simulink model "Final_Project_2_test"  (R2023b)
settings: Solver=FixedStepAuto  StartTime=0.0  StopTime=inf  FixedStep=0.01  RelTol=1e-3  EnableMultiTasking=on
libraries: arduinolib x9, arduinosensorlib x1
settings Model: ExtModeTrigDuration=2  Creator=FM23  LastModifiedBy=FM23
settings OptimizationCC: EnhancedBackFolding=on  PassReuseOutputArgsAs=Individual arguments  ZeroExternalMemoryAtStartup=off  ZeroInternalMemoryAtStartup=off  MaxStackSize=64  OptimizeBlockOrder=speed  DifferentSizesBufferReuse=on  OptimizationCustomize=off  EfficientTunableParamExpr=on
settings DebuggingCC: ParameterTunabilityLossMsg=error
settings HardwareCC: ProdBitPerInt=16  ProdBitPerPointer=16  ProdBitPerSizeT=16  ProdBitPerPtrDiffT=16  ProdLargestAtomicFloat=None  ProdWordSize=8  ProdHWDeviceType=Atmel->AVR
settings SFSimCC: MATLABDynamicMemAlloc=off
settings RTWCC: Description=Embedded Coder  SystemTargetFile=ert.tlc  HardwareBoard=Arduino Mega 2560  TemplateMakefile=ert_default_tmf  Toolchain=Arduino AVR  BuildConfiguration=Faster Runs
settings CodeAppCC: ForceParamTrailComments=on  IgnoreCustomStorageClasses=off  OperatorAnnotations=on  SimulinkDataObjDesc=on  SFDataObjDesc=on  InsertBlockDesc=on
settings ERTTargetCC: SupportContinuousTime=on  SupportVariableSizeSignals=on  ExtModeTransport=3  ExtModeStaticAlloc=on  ExtModeAutomaticAllocSize=off  ExtModeStaticAllocSize=2048  ExtModeMexFile=ext_xcp  ExtModeIntrfLevel=Level2 - Open

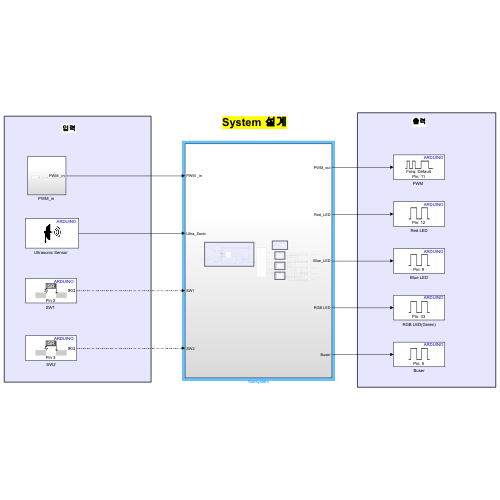
[thumbnail: Simulink's stored preview of the top-level diagram]
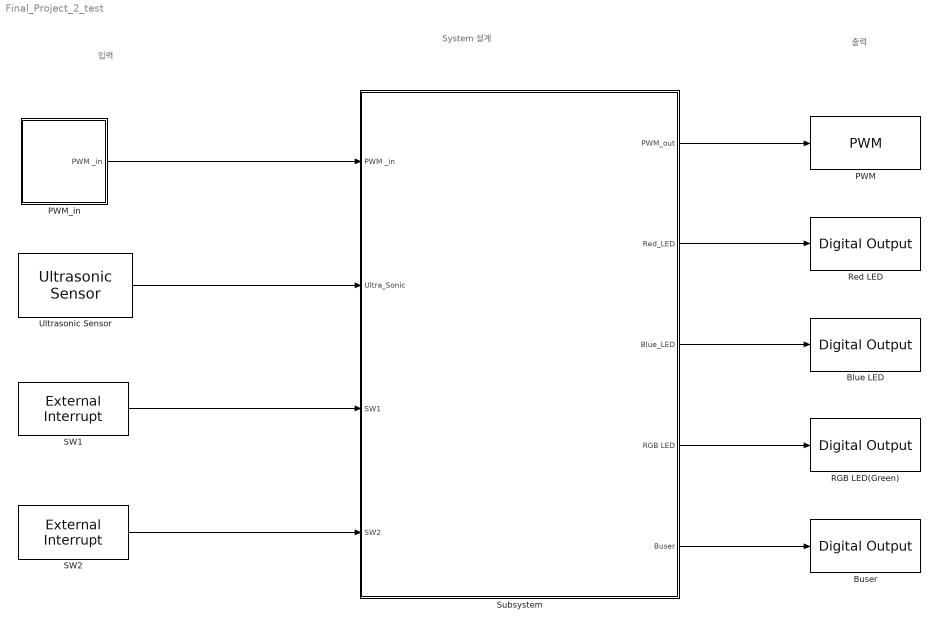
== system Final_Project_2_test ==
  note: System 설계
  note: 입력
  note: 출력
  Blue LED : arduinolib/Digital Output  pinNumber=9  Direction=output  blockPlatform=arduino
  Buser : arduinolib/Digital Output  pinNumber=5  Direction=output  blockPlatform=arduino
  "PWM  " : arduinolib/PWM  pinNumber=11  frequencyType=Default  desiredFrequency=490.2  achievableFrequency=490.2
  "PWM_in " : Subsystem
  RGB LED(Green) : arduinolib/Digital Output  pinNumber=33  Direction=output  blockPlatform=arduino
  Red LED : arduinolib/Digital Output  pinNumber=12  Direction=output  blockPlatform=arduino
  "SW1 " : arduinolib/External Interrupt  Pin=2  PullUp=off  Mode=RISING  InterruptSimulationInput=off
  SW2 : arduinolib/External Interrupt  Pin=3  PullUp=off  Mode=RISING  InterruptSimulationInput=off
  Subsystem : Subsystem
  "Ultrasonic Sensor  " : arduinosensorlib/Ultrasonic Sensor  NumSignalPins=2  TrigPin=50  EchoPin=51  SignalPin=3  SampleTime_=0.01  blockPlatform=ARDUINO
  wires:
  Subsystem/1(" PWM_out") -> "PWM  "/1
  Subsystem/2(Red_LED) -> Red LED/1
  Subsystem/3(Blue_LED) -> Blue LED/1
  "PWM_in "/1(PWM _in) -> Subsystem/1(PWM _in)
  "SW1 "/1 -> Subsystem/3(SW1)
  SW2/1 -> Subsystem/4(SW2)
  "Ultrasonic Sensor  "/1 -> Subsystem/2(Ultra_Sonic)
  Subsystem/4(RGB LED) -> RGB LED(Green)/1
  Subsystem/5(Buser) -> Buser/1

== system Final_Project_2_test/PWM_in  ==
  Analog Input1 : arduinolib/Analog Input  pinNumber=4  ReadResultsOnly=off  ConversionTriggerSource=Software  ExternalTriggerType=uint32( 0 )  OutputDataType=uint16  EnableConversionCompleteNotify=off  EnableOuputStatus=off  SampleTime=-1  blockPlatform=arduino
  Data Type Conversion : DataTypeConversion  OutDataTypeStr=uint8  SaturateOnIntegerOverflow=off  RndMeth=Floor
  Display Status : Display
  Gain : Gain  Gain=0.25
  PWM _in : Outport
  wires:
  Analog Input1/1 -> Gain/1
  Gain/1 -> Data Type Conversion/1
  Data Type Conversion/1 -> PWM _in/1, Display Status/1

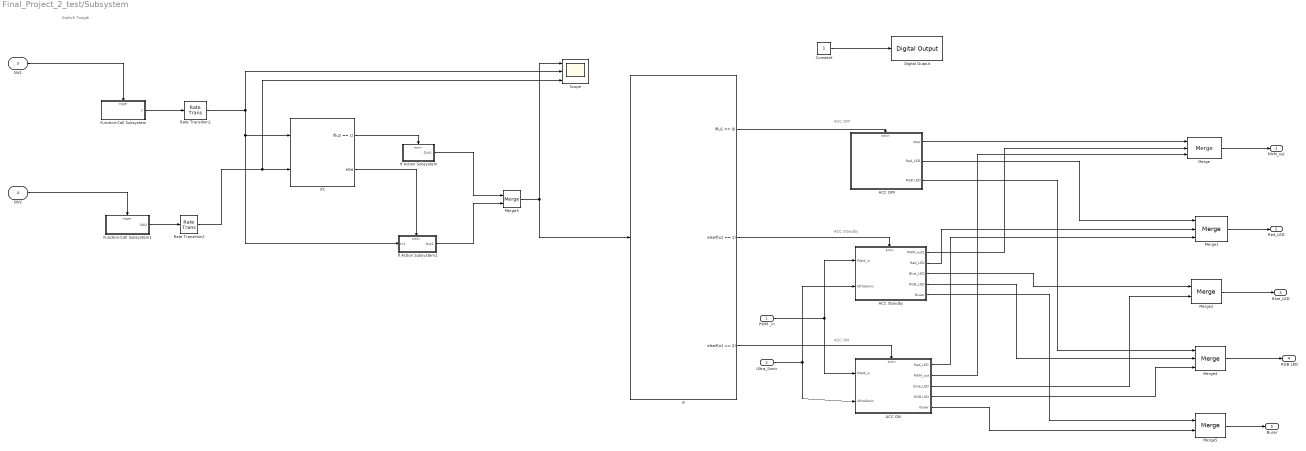
== system Final_Project_2_test/Subsystem ==
  note: ACC ON
  note: ACC standby
  note: ACC OFF
  note: Swiitch Toogle
  PWM _in : Inport
  Ultra_Sonic : Inport  Port=2
  SW1 : Inport  Port=3
  SW2 : Inport  Port=4
  ACC OFF : Subsystem  TreatAsAtomicUnit=on
  ACC ON : Subsystem  TreatAsAtomicUnit=on
  "ACC Standby   " : Subsystem  TreatAsAtomicUnit=on
  Constant : Constant
  Digital Output : arduinolib/Digital Output  pinNumber=13  Direction=output  blockPlatform=arduino
  Function-Call Subsystem : Subsystem  TreatAsAtomicUnit=on
  Function-Call Subsystem1 : Subsystem  TreatAsAtomicUnit=on
  If : If  IfExpression=u1 == 0  ElseIfExpressions=u1 == 1, u1 == 2  ShowElse=off
  If Action Subsystem : Subsystem  TreatAsAtomicUnit=on
  If Action Subsystem1 : Subsystem  TreatAsAtomicUnit=on
  If1 : If  NumInputs=2  IfExpression=u2 == 1
  Merge : Merge  Inputs=3
  Merge1 : Merge  Inputs=3
  Merge2 : Merge
  Merge3 : Merge
  Merge4 : Merge  Inputs=3
  Merge5 : Merge
  Rate Transition1 : RateTransition  Integrity=off
  Rate Transition2 : RateTransition  Integrity=off
  Scope : Scope  NumInputPorts=3
  " PWM_out" : Outport
  Red_LED : Outport  Port=2
  Blue_LED : Outport  Port=3
  RGB LED : Outport  Port=4
  Buser : Outport  Port=5
  wires:
  Function-Call Subsystem/1(y) -> Rate Transition1/1
  "ACC Standby   "/1(PWM_out2) -> Merge/2
  "ACC Standby   "/3(Blue_LED) -> Merge2/1
  If/1 -> ACC OFF/Action
  ACC ON/2(PWM_out) -> Merge/3
  ACC OFF/2(Red_LED) -> Merge1/1
  Ultra_Sonic/1 -> "ACC Standby   "/2(UltraSonic), ACC ON/2(UltraSonic)
  Rate Transition1/1 -> If Action Subsystem1/1(In1), If1/1, Scope/2
  SW1/1 -> Function-Call Subsystem/Trigger
  If/3 -> ACC ON/Action
  Merge/1 -> " PWM_out"/1
  "ACC Standby   "/2(Red_LED) -> Merge1/2
  PWM _in/1 -> "ACC Standby   "/1(PWM_in), ACC ON/1(PWM_in)
  Constant/1 -> Digital Output/1
  Merge2/1 -> Blue_LED/1
  If Action Subsystem/1(Out1) -> Merge3/1
  If1/2 -> If Action Subsystem1/Action
  ACC OFF/1(stop) -> Merge/1
  SW2/1 -> Function-Call Subsystem1/Trigger
  If Action Subsystem1/1(Out1) -> Merge3/2
  Function-Call Subsystem1/1(SW2) -> Rate Transition2/1
  Merge1/1 -> Red_LED/1
  Rate Transition2/1 -> Scope/3, If1/2
  Merge3/1 -> Scope/1, If/1
  If1/1 -> If Action Subsystem/Action
  ACC ON/3(Blue_LED) -> Merge2/2
  ACC ON/1(Red_LED) -> Merge1/3
  If/2 -> "ACC Standby   "/Action
  ACC OFF/3(RGB LED) -> Merge4/1
  "ACC Standby   "/4(RGB_LED) -> Merge4/2
  ACC ON/4(RGB LED) -> Merge4/3
  Merge4/1 -> RGB LED/1
  "ACC Standby   "/5(Buser) -> Merge5/1
  ACC ON/5(Buser) -> Merge5/2
  Merge5/1 -> Buser/1

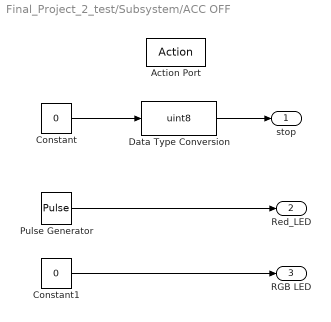
== system Final_Project_2_test/Subsystem/ACC OFF ==
  Action Port : ActionPort  ActionPortLabel=if(u1 == 0)
  Constant : Constant  Value=0
  Constant1 : Constant  Value=0
  Data Type Conversion : DataTypeConversion  OutDataTypeStr=uint8  SaturateOnIntegerOverflow=off  RndMeth=Floor
  Pulse Generator : DiscretePulseGenerator  PulseType=Time based  Period=0.4  PulseWidth=50
  stop : Outport
  Red_LED : Outport  Port=2
  RGB LED : Outport  Port=3
  wires:
  Pulse Generator/1 -> Red_LED/1
  Constant/1 -> Data Type Conversion/1
  Data Type Conversion/1 -> stop/1
  Constant1/1 -> RGB LED/1

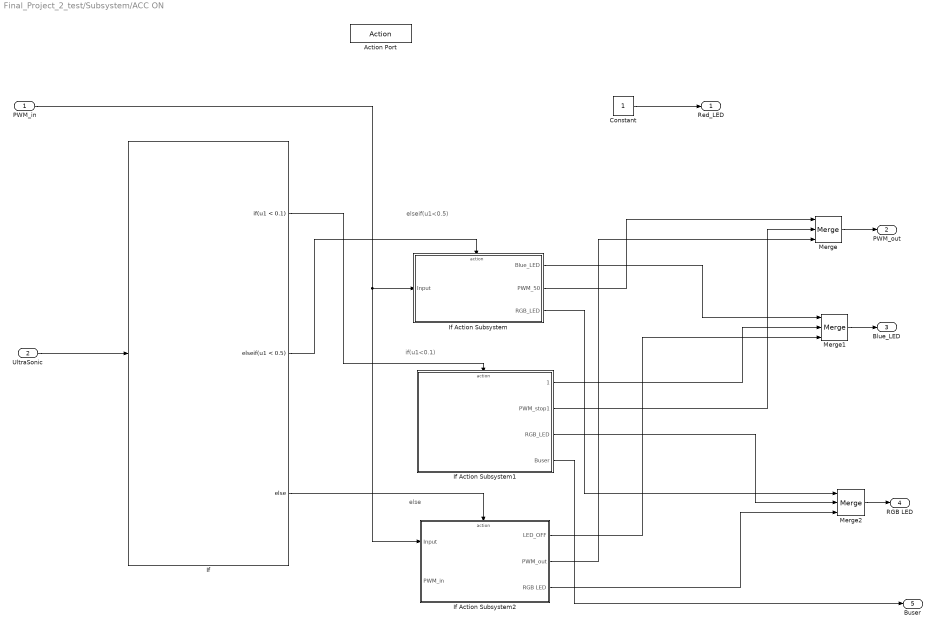
== system Final_Project_2_test/Subsystem/ACC ON ==
  note: if(u1<0.1)
  note: elseif(u1<0.5)
  note: else
  PWM_in : Inport
  UltraSonic : Inport  Port=2
  Action Port : ActionPort  ActionPortLabel=elseif( u1 == 2)
  Constant : Constant
  If : If  IfExpression=u1 < 0.1  ElseIfExpressions=u1 < 0.5
  If Action Subsystem : Subsystem  TreatAsAtomicUnit=on
  If Action Subsystem1 : Subsystem  TreatAsAtomicUnit=on
  If Action Subsystem2 : Subsystem  TreatAsAtomicUnit=on
  Merge : Merge  Inputs=3
  Merge1 : Merge  Inputs=3
  Merge2 : Merge  Inputs=3
  Red_LED : Outport
  PWM_out : Outport  Port=2  OutDataTypeStr=uint8
  Blue_LED : Outport  Port=3
  RGB LED : Outport  Port=4
  Buser : Outport  Port=5
  wires:
  If Action Subsystem2/1(LED_OFF) -> Merge1/3
  If Action Subsystem1/2(PWM_stop1) -> Merge/2
  If Action Subsystem2/2(PWM_out) -> Merge/3
  Merge1/1 -> Blue_LED/1
  If Action Subsystem/1(Blue_LED) -> Merge1/1
  If/2 -> If Action Subsystem/Action
  If/3 -> If Action Subsystem2/Action
  If Action Subsystem1/1(1) -> Merge1/2
  If Action Subsystem/2(PWM_50) -> Merge/1
  If/1 -> If Action Subsystem1/Action
  UltraSonic/1 -> If/1
  Merge/1 -> PWM_out/1
  Constant/1 -> Red_LED/1
  PWM_in/1 -> If Action Subsystem2/1(Input), If Action Subsystem/1(Input)
  If Action Subsystem/3(RGB_LED) -> Merge2/1
  If Action Subsystem1/3(RGB_LED) -> Merge2/2
  If Action Subsystem2/3(RGB LED) -> Merge2/3
  Merge2/1 -> RGB LED/1
  If Action Subsystem1/4(Buser) -> Buser/1

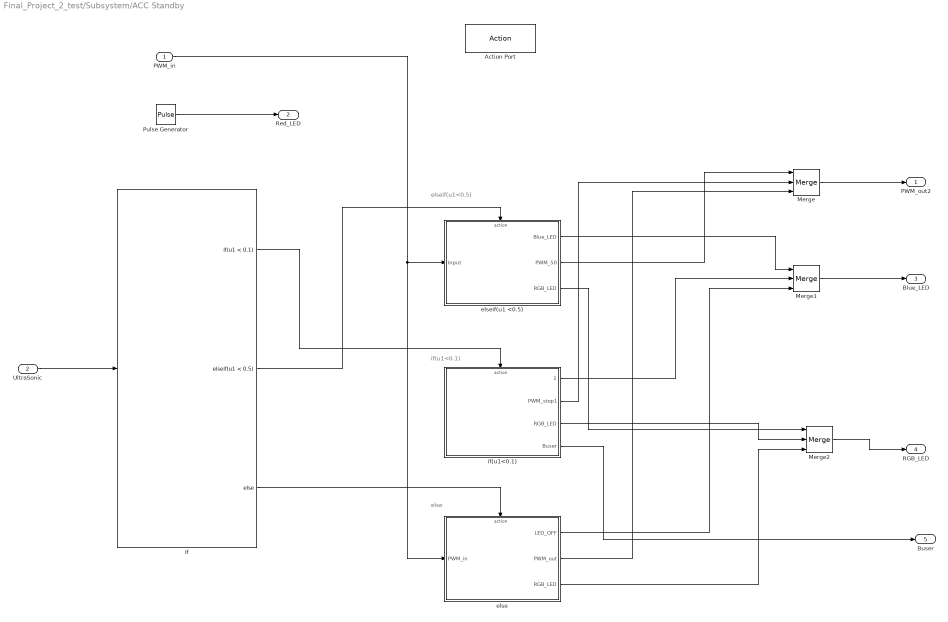
== system Final_Project_2_test/Subsystem/ACC Standby    ==
  note: else
  note: if(u1<0.1)
  note: elseif(u1<0.5)
  PWM_in : Inport  OutDataTypeStr=uint8
  UltraSonic : Inport  Port=2
  Action Port : ActionPort  ActionPortLabel=elseif(u1 == 1)
  If : If  IfExpression=u1 < 0.1  ElseIfExpressions=u1 < 0.5
  Merge : Merge  Inputs=3
  Merge1 : Merge  Inputs=3
  Merge2 : Merge  Inputs=3
  Pulse Generator : DiscretePulseGenerator  PulseType=Time based  Period=10  PulseWidth=5
  else : Subsystem  TreatAsAtomicUnit=on
  elseif(u1 <0.5) : Subsystem  TreatAsAtomicUnit=on
  if(u1<0.1) : Subsystem  TreatAsAtomicUnit=on
  PWM_out2 : Outport
  Red_LED : Outport  Port=2
  Blue_LED : Outport  Port=3
  RGB_LED : Outport  Port=4
  Buser : Outport  Port=5
  wires:
  Pulse Generator/1 -> Red_LED/1
  UltraSonic/1 -> If/1
  Merge/1 -> PWM_out2/1
  Merge1/1 -> Blue_LED/1
  If/2 -> elseif(u1 <0.5)/Action
  If/1 -> if(u1<0.1)/Action
  If/3 -> else/Action
  else/2(PWM_out) -> Merge/3
  elseif(u1 <0.5)/2(PWM_50) -> Merge/1
  elseif(u1 <0.5)/1(Blue_LED) -> Merge1/1
  if(u1<0.1)/1(1) -> Merge1/2
  if(u1<0.1)/2(PWM_stop1) -> Merge/2
  else/1(LED_OFF) -> Merge1/3
  PWM_in/1 -> else/1(PWM_in), elseif(u1 <0.5)/1(Input)
  elseif(u1 <0.5)/3(RGB_LED) -> Merge2/1
  if(u1<0.1)/3(RGB_LED) -> Merge2/2
  else/3(RGB_LED) -> Merge2/3
  Merge2/1 -> RGB_LED/1
  if(u1<0.1)/4(Buser) -> Buser/1

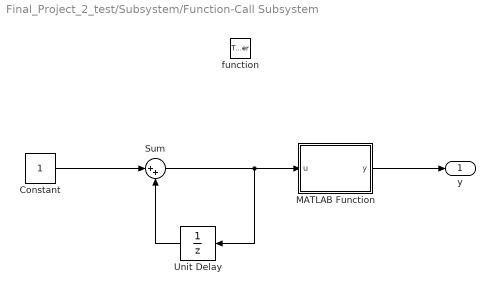
== system Final_Project_2_test/Subsystem/Function-Call Subsystem ==
  function : TriggerPort  TriggerType=function-call  VariantControl=(inherit)
  Constant : Constant
  MATLAB Function : MATLAB Function  TreatAsAtomicUnit=on
  Sum : Sum  Inputs=|++
  Unit Delay : UnitDelay  SampleTime=-1  HasFrameUpgradeWarning=on
  y : Outport
  wires:
  Constant/1 -> Sum/1
  Unit Delay/1 -> Sum/2
  Sum/1 -> Unit Delay/1, MATLAB Function/1(u)
  MATLAB Function/1(y) -> y/1

== system Final_Project_2_test/Subsystem/Function-Call Subsystem1 ==
  function : TriggerPort  TriggerType=function-call  VariantControl=(inherit)
  Constant : Constant
  MATLAB Function : MATLAB Function  TreatAsAtomicUnit=on
  Sum : Sum  Inputs=|++
  Unit Delay : UnitDelay  SampleTime=-1  HasFrameUpgradeWarning=on
  SW2 : Outport
  wires:
  Constant/1 -> Sum/1
  MATLAB Function/1(y) -> SW2/1
  Unit Delay/1 -> Sum/2
  Sum/1 -> Unit Delay/1, MATLAB Function/1(u)

== system Final_Project_2_test/Subsystem/If Action Subsystem ==
  Action Port : ActionPort  ActionPortLabel=if(u2 == 1)
  Constant : Constant  Value=0
  Out1 : Outport
  wires:
  Constant/1 -> Out1/1

== system Final_Project_2_test/Subsystem/If Action Subsystem1 ==
  In1 : Inport
  Action Port : ActionPort  ActionPortLabel=else
  Out1 : Outport
  wires:
  In1/1 -> Out1/1

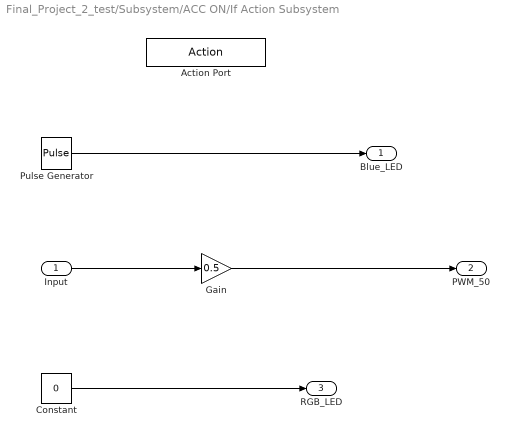
== system Final_Project_2_test/Subsystem/ACC ON/If Action Subsystem ==
  Input : Inport  OutDataTypeStr=uint8
  Action Port : ActionPort  ActionPortLabel=elseif(u1 < 0.5)
  Constant : Constant  Value=0  OutDataTypeStr=double
  Gain : Gain  Gain=0.5  OutDataTypeStr=uint8
  Pulse Generator : DiscretePulseGenerator  PulseType=Time based  Period=0.4  PulseWidth=50
  Blue_LED : Outport
  PWM_50 : Outport  Port=2  OutDataTypeStr=uint8
  RGB_LED : Outport  Port=3  OutDataTypeStr=double
  wires:
  Input/1 -> Gain/1
  Gain/1 -> PWM_50/1
  Pulse Generator/1 -> Blue_LED/1
  Constant/1 -> RGB_LED/1

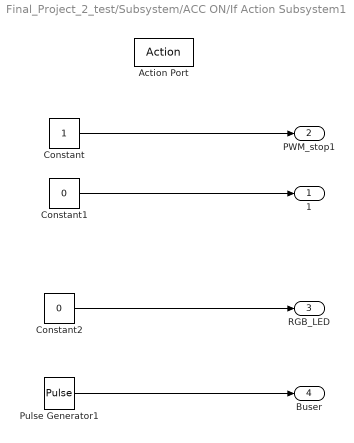
== system Final_Project_2_test/Subsystem/ACC ON/If Action Subsystem1 ==
  Action Port : ActionPort  ActionPortLabel=if(u1 < 0.1)
  Constant : Constant  OutDataTypeStr=uint8
  Constant1 : Constant  Value=0
  Constant2 : Constant  Value=0  OutDataTypeStr=double
  Pulse Generator1 : DiscretePulseGenerator  PulseType=Time based  Period=0.5  PulseWidth=50
  1 : Outport
  PWM_stop1 : Outport  Port=2  OutDataTypeStr=uint8
  RGB_LED : Outport  Port=3  OutDataTypeStr=double
  Buser : Outport  Port=4  OutDataTypeStr=double
  wires:
  Constant/1 -> PWM_stop1/1
  Constant1/1 -> 1/1
  Constant2/1 -> RGB_LED/1
  Pulse Generator1/1 -> Buser/1

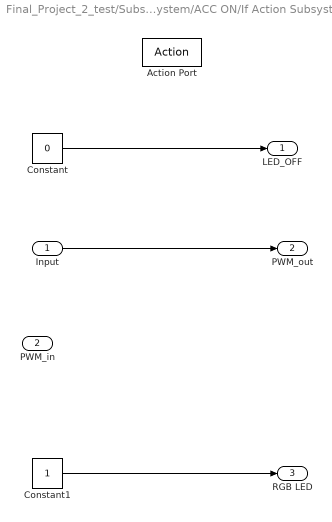
== system Final_Project_2_test/Subsystem/ACC ON/If Action Subsystem2 ==
  Input : Inport  OutDataTypeStr=uint8
  PWM_in : Inport  Port=2
  Action Port : ActionPort  ActionPortLabel=else
  Constant : Constant  Value=0
  Constant1 : Constant
  LED_OFF : Outport
  PWM_out : Outport  Port=2  OutDataTypeStr=uint8
  RGB LED : Outport  Port=3
  wires:
  Constant/1 -> LED_OFF/1
  Input/1 -> PWM_out/1
  Constant1/1 -> RGB LED/1

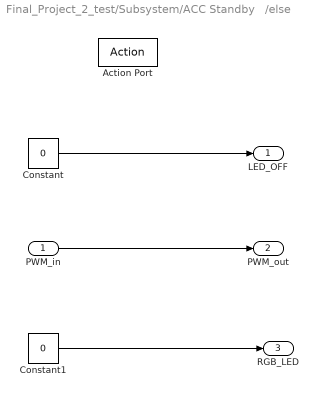
== system Final_Project_2_test/Subsystem/ACC Standby   /else ==
  PWM_in : Inport
  Action Port : ActionPort  ActionPortLabel=else
  Constant : Constant  Value=0
  Constant1 : Constant  Value=0  OutDataTypeStr=double
  LED_OFF : Outport
  PWM_out : Outport  Port=2
  RGB_LED : Outport  Port=3  OutDataTypeStr=double
  wires:
  Constant/1 -> LED_OFF/1
  PWM_in/1 -> PWM_out/1
  Constant1/1 -> RGB_LED/1

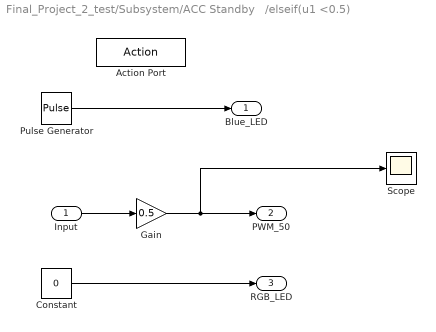
== system Final_Project_2_test/Subsystem/ACC Standby   /elseif(u1 <0.5) ==
  Input : Inport  OutDataTypeStr=uint8
  Action Port : ActionPort  ActionPortLabel=elseif(u1 < 0.5)
  Constant : Constant  Value=0  OutDataTypeStr=double
  Gain : Gain  Gain=0.5  ParamDataTypeStr=uint8  OutDataTypeStr=uint8
  Pulse Generator : DiscretePulseGenerator  PulseType=Time based  Period=0.4  PulseWidth=50
  Scope : Scope
  Blue_LED : Outport  OutDataTypeStr=double
  PWM_50 : Outport  Port=2  OutDataTypeStr=uint8
  RGB_LED : Outport  Port=3  OutDataTypeStr=double
  wires:
  Pulse Generator/1 -> Blue_LED/1
  Input/1 -> Gain/1
  Gain/1 -> Scope/1, PWM_50/1
  Constant/1 -> RGB_LED/1

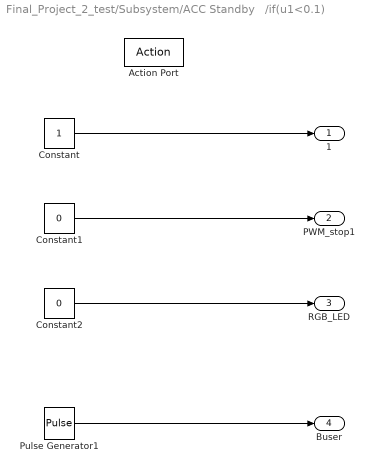
== system Final_Project_2_test/Subsystem/ACC Standby   /if(u1<0.1) ==
  Action Port : ActionPort  ActionPortLabel=if(u1 < 0.1)
  Constant : Constant  OutDataTypeStr=double
  Constant1 : Constant  Value=0  OutDataTypeStr=uint8
  Constant2 : Constant  Value=0  OutDataTypeStr=double
  Pulse Generator1 : DiscretePulseGenerator  PulseType=Time based  Period=1  PulseWidth=50
  1 : Outport  OutDataTypeStr=double
  PWM_stop1 : Outport  Port=2  OutDataTypeStr=uint8
  RGB_LED : Outport  Port=3  OutDataTypeStr=double
  Buser : Outport  Port=4  OutDataTypeStr=double
  wires:
  Constant/1 -> 1/1
  Constant1/1 -> PWM_stop1/1
  Constant2/1 -> RGB_LED/1
  Pulse Generator1/1 -> Buser/1

== matlab function Final_Project_2_test/Subsystem/Function-Call Subsystem1/MATLAB Function ==
  data: u input; y output
function y = fcn(u)
 if u > 100
     u = 1; % 여기서도 u를 재정의합니다
 end

 rem = mod(u,2);
 if rem == 0
     y = 0;
 else
     y = 1;
 end

== matlab function Final_Project_2_test/Subsystem/Function-Call Subsystem/MATLAB Function ==
  data: u input; y output
function y = fcn(u)
 if u > 100
     u = 1; % 여기서 u를 재정의합니다
 end

 rem = mod(u,3);
 if rem == 0
     y = 0;
 elseif rem == 1
     y = 1;
 else 
     y = 2;
 end
